simulink model "sldemo_hydrod"  (R2022b)
settings: Solver=ode45  StartTime=0.0  StopTime=0.1  RelTol=1e-3  AbsTol=1e-6
model workspace (MATLAB code in the model file):
  | % Load the initial conditions and initialization data
  | % Using the same MAT file as
  | % sldemo_hydcyl
  | % sldemo_hydcyl4
  | % sldemo_hydrod
  | 
  | load sldemo_hydcyl_data;
undefined symbols (not defined in the file or in its folder): Ac, C2, I, L, M, Qmax
libraries: hydlib x4, simulink x2
(part 1 of 2)
Description:
  | Two Cylinder Model with Load Constraints
  | 
  | In this model, a rigid rod supporting a large mass interconnects two
  | hydraulic actuators. The model eliminates the springs as it applies the
  | piston forces directly to the load. These forces balance the
  | gravitational force and result in both linear and rotational displacement.
  | See two related demos that use the same basic components:
  | 
  | * four cylinder model: sldemo_hydcyl4
  | * single cylinder model: sldemo_hydcyl
settings Model: PacingRate=0.010000  Creator=The MathWorks, Inc.  LastModifiedBy=The MathWorks, Inc.
settings SolverCC: AutoScaleAbsTol=off  AlgebraicLoopSolver=TrustRegion
settings DataIOCC: SaveFormat=Structure  SaveOutput=off  SaveState=on  SaveTime=off  SignalLoggingName=sldemo_hydrod_output
settings OptimizationCC: BlockReduction=off  BooleanDataType=off  ExpressionDepthLimit=2147483647  InitFltsAndDblsToZero=on  LifeSpan=inf  BufferReusableBoundary=off
settings DebuggingCC: AlgebraicLoopMsg=none  SaveWithParameterizedLinksMsg=none  UnderspecifiedInitializationDetection=Classic  MergeDetectMultiDrivingBlocksExec=none  SignalResolutionControl=TryResolveAllWithWarning  MultiTaskDSMMsg=warning  MultiTaskCondExecSysMsg=none  SigSpecEnsureSampleTimeMsg=none  IntegerOverflowMsg=none  FcnCallInpInsideContextMsg=warning  UnconnectedInputMsg=warning  UnconnectedOutputMsg=warning  UnconnectedLineMsg=warning  BusObjectLabelMismatch=none  StateNameClashWarn=warning  SFUnexpectedBacktrackingDiag=warning  SFNoUnconditionalDefaultTransitionDiag=warning  SFExecutionAtInitializationDiag=none  SFMachineParentedDataDiag=warning  IntegerSaturationMsg=none  ArithmeticOperatorsInVariantConditions=warning
settings HardwareCC: ProdBitPerPointer=32  ProdBitPerSizeT=32  ProdBitPerPtrDiffT=32  ProdLargestAtomicFloat=None  ProdIntDivRoundTo=Undefined  ProdEndianess=Unspecified  ProdWordSize=32  ProdHWDeviceType=32-bit Generic  TargetUnknown=on
settings ModelReferenceCC: EnableRefExpFcnMdlSchedulingChecks=on  PropagateSignalLabelsOutOfModel=off
settings SFSimCC: SimUseLocalCustomCode=off  CustomCodeUndefinedFunction=UseInterfaceOnly
settings RTWCC: RTWUseLocalCustomCode=off  DLArmComputeVersion=19.05
settings CodeAppCC: StateflowObjectComments=on
settings GRTTargetCC: TargetFcnLib=ansi_tfl_tmw.mat  TargetLangStandard=C89/C90 (ANSI)  CombineOutputUpdateFcns=off  GRTInterface=on
settings ConfigComp: CovMetricSettings=d  CovSaveCumulativeToWorkspaceVar=on  CovSaveSingleToWorkspaceVar=on  CovExternalEMLEnable=off

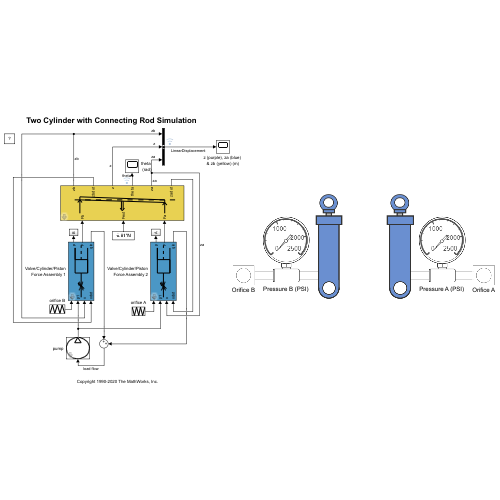
[thumbnail: Simulink's stored preview of the top-level diagram]
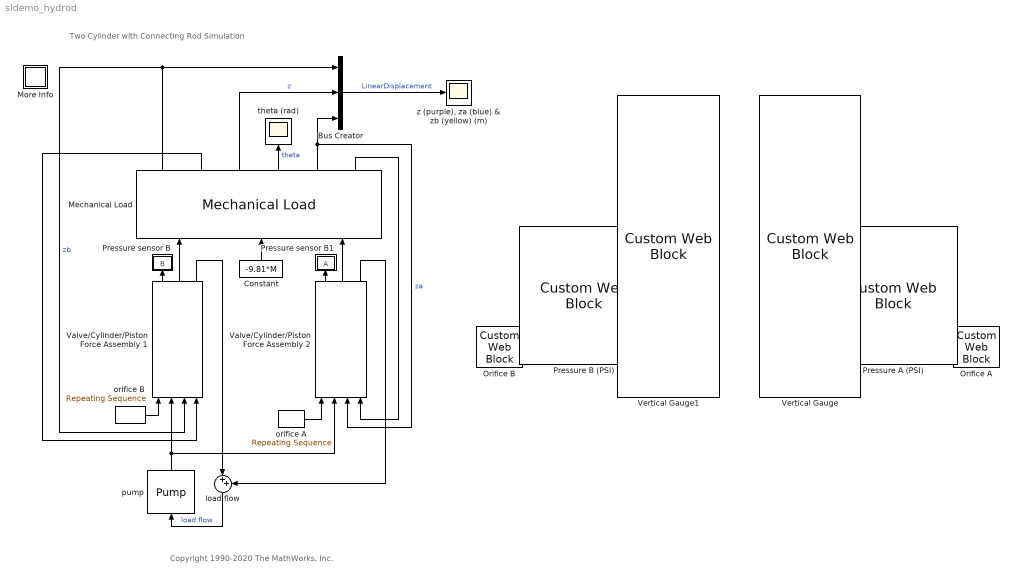
== system sldemo_hydrod ==
  note: Two Cylinder with Connecting Rod Simulation
  note: Copyright 1990-2020 The MathWorks, Inc.
  Bus Creator : BusCreator  Inputs=3
  Constant : Constant  Value=-9.81*M
  Mechanical Load : hydlib/Mechanical Load  L=L  M=M  I=I  zDotName=velocity  zName=displacement  thetaDotName=angular_velocity  thetaName=angular_displacement
  More Info : Subsystem
      settings: OpenFcn=showExample('simulink_general/sldemo_hydrodExample')
      mask Display: disp('?')
  Orifice A : CustomWebBlock  LabelPosition=Hide  ShowInitialText=on  Configuration="{\"type\":\"LinearGauge\",\"settings\":{\"BindingType\":\"signal\",\"aspectRatio\":0.2647058823529412,\"fixedAspectRatio\":\"off\",\"orientation\":\"vertical\",\"value\":0},\"components\":[{\"name\":\"LinearScaleComponent\",\"settings\":{\"bounds\":{\"max\":0.00001,\"min\":0,\"tickInterval\":\"auto\"},\"internalTickHeightScaleFactor\":0.5,\"labelColor\":[250,245,199],\"labelFont\":{\"font\":\"Arial\",\"fontSize\":12},\"labelTransparency\":0,\"needleImage\":{\"size\":[0,0],\"src\":\"\",\"srcOrientation\":\"Right\"},\"needleOffset\":[0,0],\"needleSize\":{\"height\":0,\"width\":0},\"position\":[0.036458333333333336,0.0695754716981132,3.4033018867924527,0.919921875],\"scaleColors\":[],\"scaleColorsSize\":0.2,\"showLabels\":1,\"showMinorTicks\":0,\"showSpanLine\":1,\"showTicks\":1,\"tickColor\":[250,245,200],\"tickTransparency\":0,\"valueBarColor\":[0,0,0],\"valueBarOffset\":0,\"valueBarSize\":0.23,\"valueBarTransparency\":1,\"scaleDirection\":\"BT\",\"referencePoint\":\"auto\",\"labelOffset\":0.05}},{\"name\":\"BackgroundImageComponent\",\"settings\":{\"image\":{\"size\":[0,0],\"src\":\"default\",\"srcOrientation\":null},\"position\":[0,0,1,1],\"scaleMode\":\"0\"}},{\"name\":\"ForegroundImageComponent\",\"settings\":{\"image\":{\"size\":[35,31],\"src\":\"data:image/png;base64,iVBORw0KGgoAAAANSUhEUgAAAp0AAAJbCAYAAACmZC+XAAAACXBIWXMAAA7EAAAOxAGVKw4bAAAAB3RJTUUH5AoDETghXxYhmQAAIABJREFUeJzs3XtwVeW9//HPLqBEKwRNuA3BpAoElJsBArEmgtwsRUkEWqiECug0iMgPM8Fr05wZR0+agwoRLEoqwRJFIKnIMQGEBksgQORmuWMiMFwEJWBruMX1+4OSAzZr7Z2w98rea79fM4xOnmctvtOa/Xz291kXl2EYhgAAAAAf+klDFwAAAADnI3QCAADA5widAAAA8DlCJwAAAHyO0AkAAACfI3QCAADA5widAAAA8DlCJwAAAHyu8fUc7HK5vFUHAAAAAkR93i1EpxMAAAA+R+gEAACAzxE6AQAA ...(+26324 chars)\",\"srcOrientation\":\"vertical\"},\"isForeground\":1,\"position\":[0,0,1,1],\"scaleMode\":\"0\"}}]}"
  Orifice B : CustomWebBlock  LabelPosition=Hide  ShowInitialText=on  Configuration="{\"type\":\"LinearGauge\",\"settings\":{\"BindingType\":\"signal\",\"aspectRatio\":0.2647058823529412,\"fixedAspectRatio\":\"off\",\"orientation\":\"vertical\",\"value\":0},\"components\":[{\"name\":\"LinearScaleComponent\",\"settings\":{\"bounds\":{\"max\":0.00001,\"min\":0,\"tickInterval\":\"auto\"},\"internalTickHeightScaleFactor\":0.5,\"labelColor\":[250,245,199],\"labelFont\":{\"font\":\"Arial\",\"fontSize\":12},\"labelTransparency\":0,\"needleImage\":{\"size\":[0,0],\"src\":\"\",\"srcOrientation\":\"Right\"},\"needleOffset\":[0,0],\"needleSize\":{\"height\":0,\"width\":0},\"position\":[0.036458333333333336,0.0695754716981132,3.4033018867924527,0.919921875],\"scaleColors\":[],\"scaleColorsSize\":0.2,\"showLabels\":1,\"showMinorTicks\":0,\"showSpanLine\":1,\"showTicks\":1,\"tickColor\":[250,245,200],\"tickTransparency\":0,\"valueBarColor\":[0,0,0],\"valueBarOffset\":0,\"valueBarSize\":0.23,\"valueBarTransparency\":1,\"scaleDirection\":\"BT\",\"referencePoint\":\"auto\",\"labelOffset\":0.05}},{\"name\":\"BackgroundImageComponent\",\"settings\":{\"image\":{\"size\":[0,0],\"src\":\"default\",\"srcOrientation\":null},\"position\":[0,0,1,1],\"scaleMode\":\"0\"}},{\"name\":\"ForegroundImageComponent\",\"settings\":{\"image\":{\"size\":[35,31],\"src\":\"data:image/png;base64,iVBORw0KGgoAAAANSUhEUgAAAp0AAAJbCAYAAACmZC+XAAAACXBIWXMAAA7EAAAOxAGVKw4bAAAAB3RJTUUH5AoDETghXxYhmQAAIABJREFUeJzs3XtwVeW9//HPLqBEKwRNuA3BpAoElJsBArEmgtwsRUkEWqiECug0iMgPM8Fr05wZR0+agwoRLEoqwRJFIKnIMQGEBksgQORmuWMiMFwEJWBruMX1+4OSAzZr7Z2w98rea79fM4xOnmctvtOa/Xz291kXl2EYhgAAAAAf+klDFwAAAADnI3QCAADA5widAAAA8DlCJwAAAHyO0AkAAACfI3QCAADA5widAAAA8DlCJwAAAHyu8fUc7HK5vFUHAAAAAkR93i1EpxMAAAA+R+gEAACAzxE6AQAA ...(+26324 chars)\",\"srcOrientation\":\"vertical\"},\"isForeground\":1,\"position\":[0,0,1,1],\"scaleMode\":\"0\"}}]}"
  Pressure A (PSI) : CustomWebBlock  LabelPosition=Hide  ShowInitialText=on  Configuration="{\"type\":\"CircularGauge\",\"settings\":{\"BindingType\":\"signal\",\"aspectRatio\":0.9677819083023544,\"direction\":\"cw\",\"fixedAspectRatio\":\"on\",\"flipLimits\":0,\"orientation\":\"horizontal\",\"value\":0,\"backgroundOffset\":0.14},\"components\":[{\"name\":\"CircularScaleComponent\",\"settings\":{\"bounds\":{\"max\":2500,\"min\":0,\"tickInterval\":\"auto\"},\"direction\":\"cw\",\"flipLimits\":0,\"innerRadius\":0.75,\"internalTickHeightScaleFactor\":1,\"labelColor\":[38,38,38],\"labelFont\":{\"font\":\"Arial\",\"fontSize\":12},\"labelTransparency\":1,\"minorTickHeightScaleFactor\":0.2,\"needleImage\":{\"size\":[79,20],\"src\":\"data:image/svg+xml;base64,PD94bWwgdmVyc2lvbj0iMS4wIiBlbmNvZGluZz0idXRmLTgiPz4KPCEtLSBHZW5lcmF0b3I6IEFkb2JlIElsbHVzdHJhdG9yIDI0LjEuMiwgU1ZHIEV4cG9ydCBQbHVnLUluIC4gU1ZHIFZlcnNpb246IDYuMDAgQnVpbGQgMCkgIC0tPgo8c3ZnIHZlcnNpb249IjEuMSIgaWQ9IkxheWVyXzEiIHhtbG5zPSJodHRwOi8vd3d3LnczLm9yZy8yMDAwL3N2ZyIgeG1sbnM6eGxpbms9Imh0dHA6Ly93d3cudzMub3JnLzE5OTkveGxpbmsiIHg9IjBweCIgeT0iMHB4IgoJIHZpZXdCb3g9IjAgMCA3OC43IDIwIiBzdHlsZT0iZW5hYmxlLWJhY2tncm91bmQ6bmV3IDAgMCA3OC43IDIwOyIgeG1sOnNwYWNlPSJwcmVzZXJ2ZSI+CjxwYXRoIGQ9Ik01My4xLDUuOGwyNS42LTEuNGwtMy41LDVsMy4xLDUuMmwtMjUuNC0xLjNjLTEuNSwyLjMtNC4yLDMuNC02LjksM2MtMi4yLTAuMy00LjItMS43LTUuMi0zLjdMMC45LDEwLjgKCWMtMS4xLDAtMS4yLTEuNi0wLjEtMS43bDM5LjktMi43QzQyLDMuNiw0NSwyLDQ4LDIuNEM1MC4yLDIuOCw1Miw0LDUzLjEsNS44TDUzLjEsNS44eiBNNTMuNywxMS42bDIxLjQsMS4xbC0yLTMuNGwyLjEtMy4xCglMNTMuOCw3LjVDNTMuOSw4LDU0LDguNSw1NCw5LjFDNTQuMSw5LjksNTQsMTAuOCw1My43LDExLjZMNTMuNywxMS42eiBNNDAuMSw4LjJMMTkuMyw5LjVjLTMuOSwwLjMtMy45LDAuMiwwLDAuNGwyMC45LDEKCUM0MCwxMC41LDQwLDEwLDQwLDkuNUM0MCw5LjEsNDAsOC42LDQwLjEsOC4yTDQwLjEsOC4yeiBNNDcuOCw0LjFjLTMuMy0wLjUtNi4yLDIuMS02LjEsNS40YzAsMi42LDEuOSw0LjgsNC41LDUuMQoJYzMuMywwLjUsNi4zLTIuMiw2LjEtNS41QzUyLjIsNi42LDUwLjMsNC41LDQ3LjgsNC4xTDQ3LjgsNC4xeiIvPgo8L3N2Zz4K\"},\"needleOffset\":[0.061149395709068396,0],\"needleOrientation\":-45,\"needleRotation\":180,\"needleSize\":{\"height\":0.1101177838554453,\"width\":0.43719941652583294},\"outerRadius\":0.9,\"position\":[-0.001375,0.1378196848359597,0.7199690002583312,0.75],\"scaleAngle\":270,\"scaleAngleOffset\":135,\"scaleColors\":[],\"scaleColorsSize\":0.2,\"scalePosition\":[0,0,1,1],\"showLabels\":1,\"showMinorTicks\":1,\"showSpanLine\":1,\"showTicks\":1,\"tickColor\":[38,38,38],\"tickTransparency\":1,\"valueBarColor\":[0,114,189],\"valueBarPosition\":[0,0,1,1],\"valueBarSize\":0.2,\"valueBarTransparency\":0,\"scaleDirection\":\"CW\",\"referencePoint\":\"auto\",\"labelRadius\":0.528}},{\"name\":\"BackgroundImageComponent\",\"settings\":{\"image\":{\"size\":[6248,6456],\"src\":\"data:image/svg+xml;base64,PD94bWwgdmVyc2lvbj0iMS4wIiBlbmNvZGluZz0idXRmLTgiPz4KPCEtLSBHZW5lcmF0b3I6IEFkb2JlIElsbHVzdHJhdG9yIDI0LjEuMiwgU1ZHIEV4cG9ydCBQbHVnLUluIC4gU1ZHIFZlcnNpb246IDYuMDAgQnVpbGQgMCkgIC0tPgo8c3ZnIHZlcnNpb249IjEuMSIgaWQ9IkxheWVyXzEiIHhtbG5zOnhvZG09Imh0dHA6Ly93d3cuY29yZWwuY29tL2NvcmVsZHJhdy9vZG0vMjAwMyIKCSB4bWxucz0iaHR0cDovL3d3dy53My5vcmcvMjAwMC9zdmciIHhtbG5zOnhsaW5rPSJodHRwOi8vd3d3LnczLm9yZy8xOTk5L3hsaW5rIiB4 ...(+3504 chars)\",\"srcOrientation\":\"horizontal\"},\"position\":[0,0,1,1],\"scaleMode\":\"0\"}},{\"name\":\"ForegroundImageComponent\",\"settings\":{\"image\":{\"size\":[0,0],\"src\":\"default\",\"srcOrientation\":[]},\"isForeground\":1,\"position\":[0,0,1,1],\"scaleMode\":\"0\"}}]}"
  Pressure B (PSI) : CustomWebBlock  LabelPosition=Hide  ShowInitialText=on  Configuration="{\"type\":\"CircularGauge\",\"settings\":{\"BindingType\":\"signal\",\"aspectRatio\":0.9677819083023544,\"direction\":\"cw\",\"fixedAspectRatio\":\"on\",\"flipLimits\":0,\"orientation\":\"horizontal\",\"value\":0,\"backgroundOffset\":0.14},\"components\":[{\"name\":\"CircularScaleComponent\",\"settings\":{\"bounds\":{\"max\":2500,\"min\":0,\"tickInterval\":\"auto\"},\"direction\":\"cw\",\"flipLimits\":0,\"innerRadius\":0.75,\"internalTickHeightScaleFactor\":1,\"labelColor\":[38,38,38],\"labelFont\":{\"font\":\"Arial\",\"fontSize\":12},\"labelTransparency\":1,\"minorTickHeightScaleFactor\":0.2,\"needleImage\":{\"size\":[79,20],\"src\":\"data:image/svg+xml;base64,PD94bWwgdmVyc2lvbj0iMS4wIiBlbmNvZGluZz0idXRmLTgiPz4KPCEtLSBHZW5lcmF0b3I6IEFkb2JlIElsbHVzdHJhdG9yIDI0LjEuMiwgU1ZHIEV4cG9ydCBQbHVnLUluIC4gU1ZHIFZlcnNpb246IDYuMDAgQnVpbGQgMCkgIC0tPgo8c3ZnIHZlcnNpb249IjEuMSIgaWQ9IkxheWVyXzEiIHhtbG5zPSJodHRwOi8vd3d3LnczLm9yZy8yMDAwL3N2ZyIgeG1sbnM6eGxpbms9Imh0dHA6Ly93d3cudzMub3JnLzE5OTkveGxpbmsiIHg9IjBweCIgeT0iMHB4IgoJIHZpZXdCb3g9IjAgMCA3OC43IDIwIiBzdHlsZT0iZW5hYmxlLWJhY2tncm91bmQ6bmV3IDAgMCA3OC43IDIwOyIgeG1sOnNwYWNlPSJwcmVzZXJ2ZSI+CjxwYXRoIGQ9Ik01My4xLDUuOGwyNS42LTEuNGwtMy41LDVsMy4xLDUuMmwtMjUuNC0xLjNjLTEuNSwyLjMtNC4yLDMuNC02LjksM2MtMi4yLTAuMy00LjItMS43LTUuMi0zLjdMMC45LDEwLjgKCWMtMS4xLDAtMS4yLTEuNi0wLjEtMS43bDM5LjktMi43QzQyLDMuNiw0NSwyLDQ4LDIuNEM1MC4yLDIuOCw1Miw0LDUzLjEsNS44TDUzLjEsNS44eiBNNTMuNywxMS42bDIxLjQsMS4xbC0yLTMuNGwyLjEtMy4xCglMNTMuOCw3LjVDNTMuOSw4LDU0LDguNSw1NCw5LjFDNTQuMSw5LjksNTQsMTAuOCw1My43LDExLjZMNTMuNywxMS42eiBNNDAuMSw4LjJMMTkuMyw5LjVjLTMuOSwwLjMtMy45LDAuMiwwLDAuNGwyMC45LDEKCUM0MCwxMC41LDQwLDEwLDQwLDkuNUM0MCw5LjEsNDAsOC42LDQwLjEsOC4yTDQwLjEsOC4yeiBNNDcuOCw0LjFjLTMuMy0wLjUtNi4yLDIuMS02LjEsNS40YzAsMi42LDEuOSw0LjgsNC41LDUuMQoJYzMuMywwLjUsNi4zLTIuMiw2LjEtNS41QzUyLjIsNi42LDUwLjMsNC41LDQ3LjgsNC4xTDQ3LjgsNC4xeiIvPgo8L3N2Zz4K\"},\"needleOffset\":[0.061149395709068396,0],\"needleOrientation\":-45,\"needleRotation\":180,\"needleSize\":{\"height\":0.1101177838554453,\"width\":0.43719941652583294},\"outerRadius\":0.9,\"position\":[0.0065,0.1379808323486937,0.7195746356833399,0.726],\"scaleAngle\":270,\"scaleAngleOffset\":135,\"scaleColors\":[],\"scaleColorsSize\":0.2,\"scalePosition\":[0,0,1,1],\"showLabels\":1,\"showMinorTicks\":1,\"showSpanLine\":1,\"showTicks\":1,\"tickColor\":[38,38,38],\"tickTransparency\":1,\"valueBarColor\":[0,114,189],\"valueBarPosition\":[0,0,1,1],\"valueBarSize\":0.2,\"valueBarTransparency\":0,\"scaleDirection\":\"CW\",\"referencePoint\":\"auto\",\"labelRadius\":0.528}},{\"name\":\"BackgroundImageComponent\",\"settings\":{\"image\":{\"size\":[6248,6456],\"src\":\"data:image/svg+xml;base64,PD94bWwgdmVyc2lvbj0iMS4wIiBlbmNvZGluZz0idXRmLTgiPz4KPCEtLSBHZW5lcmF0b3I6IEFkb2JlIElsbHVzdHJhdG9yIDI0LjEuMiwgU1ZHIEV4cG9ydCBQbHVnLUluIC4gU1ZHIFZlcnNpb246IDYuMDAgQnVpbGQgMCkgIC0tPgo8c3ZnIHZlcnNpb249IjEuMSIgaWQ9IkxheWVyXzEiIHhtbG5zOnhvZG09Imh0dHA6Ly93d3cuY29yZWwuY29tL2NvcmVsZHJhdy9vZG0vMjAwMyIKCSB4bWxucz0iaHR0cDovL3d3dy53My5vcmcvMjAwMC9zdmciIHhtbG5zOnhsaW5rPSJodHRwOi8vd3d3LnczLm9yZy8xOTk5L3hsaW5rIiB4 ...(+3504 chars)\",\"srcOrientation\":\"horizontal\"},\"position\":[0,0,1,1],\"scaleMode\":\"0\"}},{\"name\":\"ForegroundImageComponent\",\"settings\":{\"image\":{\"size\":[0,0],\"src\":\"default\",\"srcOrientation\":[]},\"isForeground\":1,\"position\":[0,0,1,1],\"scaleMode\":\"0\"}}]}"
  Pressure sensor B : Subsystem
  Pressure sensor B1 : Subsystem
  Valve/Cylinder/Piston Force Assembly 1 : hydlib/Valve//Cylinder//Piston Force Assembly  C1=C1  Ac=Ac  Cd=Cd  rho=rho  V30=V30  beta=Beta  p30=9.81*M/2/Ac  assemblyName=forceLeft
  Valve/Cylinder/Piston Force Assembly 2 : hydlib/Valve//Cylinder//Piston Force Assembly  C1=C1  Ac=Ac  Cd=Cd  rho=rho  V30=V30  beta=Beta  p30=9.81*M/2/Ac  assemblyName=forceRight
  Vertical Gauge : CustomWebBlock  LabelPosition=Hide  ShowInitialText=on  Configuration="{\"type\":\"LinearGauge\",\"settings\":{\"BindingType\":\"signal\",\"aspectRatio\":0.3333333333333333,\"fixedAspectRatio\":\"on\",\"orientation\":\"vertical\",\"value\":0},\"components\":[{\"name\":\"LinearScaleComponent\",\"settings\":{\"bounds\":{\"max\":0.012,\"min\":0,\"tickInterval\":\"auto\"},\"internalTickHeightScaleFactor\":0.5,\"labelColor\":[250,245,199],\"labelFont\":{\"font\":\"Arial\",\"fontSize\":12},\"labelTransparency\":0,\"needleImage\":{\"size\":[192,576],\"src\":\"data:image/svg+xml;base64,PHN2ZyB3aWR0aD0iMTkyIiBoZWlnaHQ9IjU3NiIgeG1sbnM9Imh0dHA6Ly93d3cudzMub3JnLzIwMDAvc3ZnIiB4bWxuczp4bGluaz0iaHR0cDovL3d3dy53My5vcmcvMTk5OS94bGluayIgb3ZlcmZsb3c9ImhpZGRlbiI+PGRlZnM+PGNsaXBQYXRoIGlkPSJjbGlwMCI+PHBhdGggZD0iTTAgMCAxOTIgMCAxOTIgNTc2IDAgNTc2WiIgZmlsbC1ydWxlPSJldmVub2RkIiBjbGlwLXJ1bGU9ImV2ZW5vZGQiLz48L2NsaXBQYXRoPjwvZGVmcz48ZyBjbGlwLXBhdGg9InVybCgjY2xpcDApIj48cmVjdCB4PSIwIiB5PSIwIiB3aWR0aD0iMTkyIiBoZWlnaHQ9IjU3NiIgZmlsbD0iI0ZGRkZGRiIgZmlsbC1vcGFjaXR5PSIwIi8+PHJlY3QgeD0iNzkuNTAwMSIgeT0iMTIxLjUiIHdpZHRoPSIzMiIgaGVpZ2h0PSI0NTIiIHN0cm9rZT0iIzAwMDAwMCIgc3Ryb2tlLXdpZHRoPSI3IiBzdHJva2UtbWl0ZXJsaW1pdD0iOCIgZmlsbD0iI0E2QTZBNiIvPjxwYXRoIGQ9Ik00MC41MDAxIDU4QzQwLjUwMDEgMjcuOTAwNSA2NC45MDA1IDMuNTAwMDUgOTUgMy41MDAwNSAxMjUuMSAzLjUwMDA1IDE0OS41IDI3LjkwMDUgMTQ5LjUgNTggMTQ5LjUgODguMDk5NiAxMjUuMSAxMTIuNSA5NSAxMTIuNSA2NC45MDA1IDExMi41IDQwLjUwMDEgODguMDk5NiA0MC41MDAxIDU4WiIgc3Ryb2tlPSIjMDAwMDAwIiBzdHJva2Utd2lkdGg9IjUiIHN0cm9rZS1taXRlcmxpbWl0PSI4IiBmaWxsPSIjNDQ3MkM0IiBmaWxsLXJ1bGU9ImV2ZW5vZGQiLz48cmVjdCB4PSI2MS41MDAxIiB5PSIxMDEuNSIgd2lkdGg9IjY5IiBoZWlnaHQ9IjIwIiBzdHJva2U9IiMwMDAwMDAiIHN0cm9rZS13aWR0aD0iNyIgc3Ryb2tlLW1pdGVybGltaXQ9IjgiIGZpbGw9IiM0NDcyQzQiLz48cGF0aCBkPSJNNjQuNTAwMSA1NS4wMDAxQzY0LjUwMDEgMzguMTU1NCA3OC4xNTU0IDI0LjUwMDEgOTUuMDAwMSAyNC41MDAxIDExMS44NDUgMjQuNTAwMSAxMjUuNSAzOC4xNTU0IDEyNS41IDU1LjAwMDEgMTI1LjUgNzEuODQ0NyAxMTEuODQ1IDg1LjUwMDEgOTUuMDAwMSA4NS41MDAxIDc4LjE1NTQgODUuNTAwMSA2NC41MDAxIDcxLjg0NDcgNjQuNTAwMSA1NS4wMDAxWiIgc3Ryb2tlPSIjMDAwMDAwIiBzdHJva2Utd2lkdGg9IjUiIHN0cm9rZS1taXRlcmxpbWl0PSI4IiBmaWxsPSIjRkZGRkZGIiBmaWxsLXJ1bGU9ImV2ZW5vZGQiLz48L2c+PC9zdmc+\",\"srcOrientation\":\"Right\"},\"needleOffset\":[-0.0371900826446281,-0.19204801200300076],\"needleSize\":{\"height\":0.587378640776699,\"width\":0.6125919117647058},\"position\":[0.2412014563106796,0.2516084558823529,0.5994944852941176,0.39638956310679613],\"scaleColors\":[],\"scaleColorsSize\":0.2,\"showLabels\":1,\"showMinorTicks\":0,\"showSpanLine\":1,\"showTicks\":1,\"tickColor\":[250,245,200],\"tickTransparency\":0,\"valueBarColor\":[23,89,176],\"valueBarOffset\":0,\"valueBarSize\":0.23,\"valueBarTransparency\":0,\"scaleDirection\":\"BT\",\"referencePoint\":\"auto\",\"labelOffset\":0.05}},{\"name\":\"BackgroundImageComponent\",\"settings\":{\"image\":{\"size\":[0,0],\"src\":\"default\",\"srcOrientation\":null},\"position\":[0,0,1,1],\"scaleMode\":\"0\"}},{\"name\":\"ForegroundImageComponent\",\"settings\":{\"image\":{\"size\":[288,864],\"src\":\"data:image/svg+xml;base64,PHN2ZyB3aWR0aD0iMjg4IiBoZWlnaHQ9Ijg2NCIgeG1sbnM9Imh0dHA6Ly93d3cudzMub3JnLzIwMDAvc3ZnIiB4bWxuczp4bGluaz0iaHR0cDovL3d3dy53My5vcmcvMTk5OS94bGluayIgb3ZlcmZsb3c9ImhpZGRlbiI+PGRlZnM+PGNsaXBQYXRoIGlkPSJjbGlwMCI+PHBhdGggZD0iTTAgMCAyODggMCAyODggODY0IDAgODY0WiIgZmlsbC1ydWxlPSJldmVub2RkIiBjbGlwLXJ1bGU9ImV2ZW5vZGQiLz48L2NsaXBQYXRoPjwvZGVmcz48ZyBjbGlwLXBhdGg9InVybCgjY2xpcDApIj48cmVjdCB4PSIwIiB5PSIwIiB3aWR0aD0iMjg4IiBoZWlnaHQ9Ijg2NCIgZmlsbD0iI0ZGRkZGRiIgZmlsbC1vcGFjaXR5PSIwIi8+PHJlY3QgeD0iODYuNTAwMSIgeT0iNDMyLjUiIHdpZHRoPSIxMTYiIGhlaWdodD0iMzY3IiBzdHJva2U9IiMwMDAwMDAiIHN0cm9rZS13aWR0aD0iNyIgc3Ryb2tlLW1pdGVybGltaXQ9IjgiIGZpbGw9IiM0NDcyQzQiLz48cmVjdCB4PSI3Mi41MDAxIiB5PSIzODMuNSIgd2lkdGg9IjE0NiIgaGVpZ2h0PSI0OSIgc3Ryb2tlPSIjMDAwMDAwIiBzdHJva2Utd2lkdGg9IjciIHN0cm9rZS1taXRlcmxpbWl0PSI4IiBmaWxsPSIjNDQ3MkM0Ii8+PHBhdGggZD0iTTIwMi41IDc5MkMyMDIuNSA4MjMuNzU3IDE3Ni41MzMgODQ5LjUgMTQ0LjUgODQ5LjUgMTEyLjcyMSA4NDkuNSA4Ni44NTk1IDgyNC4xNDcgODYuNTAzNyA3OTIuNjQ0TDE0NC41IDc5MloiIHN0cm9rZT0iIzAwMDAwMCIgc3Ryb2tlLXdpZHRoPSI3IiBzdHJva2UtbWl0ZXJsaW1pdD0iOCIgZmlsbD0iIzQ0NzJDNCIgZmlsbC1ydWxlPSJldmVub2RkIi8+PHJlY3QgeD0iOTEiIHk9Ijc0NyIgd2lkdGg9IjEwOCIgaGVpZ2h0PSI0OSIgZmlsbD0iIzQ0NzJDNCIvPjxwYXRoIGQ9Ik0xMDkuNSA3OTEuNUMxMDkuNSA3NzEuNjE4IDEyNS42MTggNzU1LjUgMTQ1LjUgNzU1LjUgMTY1LjM4MiA3NTUuNSAxODEuNSA3NzEuNjE4IDE4MS41IDc5MS41IDE4MS41IDgxMS4zODIgMTY1LjM4MiA4MjcuNSAxNDUuNSA4MjcuNSAxMjUuNjE4IDgyNy41IDEwOS41IDgxMS4zODIgMTA5LjUgNzkxLjVaIiBzdHJva2U9IiMwMDAwMDAiIHN0cm9rZS13aWR0aD0iNSIgc3Ryb2tlLW1pdGVybGltaXQ9IjgiIGZpbGw9IiNGRkZGRkYiIGZpbGwtcnVsZT0iZXZlbm9kZCIvPjwvZz48L3N2Zz4=\",\"srcOrientation\":\"vertical\"},\"isForeground\":1,\"position\":[0,0,1,1],\"scaleMode\":\"0\"}}]}"
  Vertical Gauge1 : CustomWebBlock  LabelPosition=Hide  ShowInitialText=on  Configuration="{\"type\":\"LinearGauge\",\"settings\":{\"BindingType\":\"signal\",\"aspectRatio\":0.3333333333333333,\"fixedAspectRatio\":\"on\",\"orientation\":\"vertical\",\"value\":0},\"components\":[{\"name\":\"LinearScaleComponent\",\"settings\":{\"bounds\":{\"max\":0.012,\"min\":0,\"tickInterval\":\"auto\"},\"internalTickHeightScaleFactor\":0.5,\"labelColor\":[250,245,199],\"labelFont\":{\"font\":\"Arial\",\"fontSize\":12},\"labelTransparency\":0,\"needleImage\":{\"size\":[192,576],\"src\":\"data:image/svg+xml;base64,PHN2ZyB3aWR0aD0iMTkyIiBoZWlnaHQ9IjU3NiIgeG1sbnM9Imh0dHA6Ly93d3cudzMub3JnLzIwMDAvc3ZnIiB4bWxuczp4bGluaz0iaHR0cDovL3d3dy53My5vcmcvMTk5OS94bGluayIgb3ZlcmZsb3c9ImhpZGRlbiI+PGRlZnM+PGNsaXBQYXRoIGlkPSJjbGlwMCI+PHBhdGggZD0iTTAgMCAxOTIgMCAxOTIgNTc2IDAgNTc2WiIgZmlsbC1ydWxlPSJldmVub2RkIiBjbGlwLXJ1bGU9ImV2ZW5vZGQiLz48L2NsaXBQYXRoPjwvZGVmcz48ZyBjbGlwLXBhdGg9InVybCgjY2xpcDApIj48cmVjdCB4PSIwIiB5PSIwIiB3aWR0aD0iMTkyIiBoZWlnaHQ9IjU3NiIgZmlsbD0iI0ZGRkZGRiIgZmlsbC1vcGFjaXR5PSIwIi8+PHJlY3QgeD0iNzkuNTAwMSIgeT0iMTIxLjUiIHdpZHRoPSIzMiIgaGVpZ2h0PSI0NTIiIHN0cm9rZT0iIzAwMDAwMCIgc3Ryb2tlLXdpZHRoPSI3IiBzdHJva2UtbWl0ZXJsaW1pdD0iOCIgZmlsbD0iI0E2QTZBNiIvPjxwYXRoIGQ9Ik00MC41MDAxIDU4QzQwLjUwMDEgMjcuOTAwNSA2NC45MDA1IDMuNTAwMDUgOTUgMy41MDAwNSAxMjUuMSAzLjUwMDA1IDE0OS41IDI3LjkwMDUgMTQ5LjUgNTggMTQ5LjUgODguMDk5NiAxMjUuMSAxMTIuNSA5NSAxMTIuNSA2NC45MDA1IDExMi41IDQwLjUwMDEgODguMDk5NiA0MC41MDAxIDU4WiIgc3Ryb2tlPSIjMDAwMDAwIiBzdHJva2Utd2lkdGg9IjUiIHN0cm9rZS1taXRlcmxpbWl0PSI4IiBmaWxsPSIjNDQ3MkM0IiBmaWxsLXJ1bGU9ImV2ZW5vZGQiLz48cmVjdCB4PSI2MS41MDAxIiB5PSIxMDEuNSIgd2lkdGg9IjY5IiBoZWlnaHQ9IjIwIiBzdHJva2U9IiMwMDAwMDAiIHN0cm9rZS13aWR0aD0iNyIgc3Ryb2tlLW1pdGVybGltaXQ9IjgiIGZpbGw9IiM0NDcyQzQiLz48cGF0aCBkPSJNNjQuNTAwMSA1NS4wMDAxQzY0LjUwMDEgMzguMTU1NCA3OC4xNTU0IDI0LjUwMDEgOTUuMDAwMSAyNC41MDAxIDExMS44NDUgMjQuNTAwMSAxMjUuNSAzOC4xNTU0IDEyNS41IDU1LjAwMDEgMTI1LjUgNzEuODQ0NyAxMTEuODQ1IDg1LjUwMDEgOTUuMDAwMSA4NS41MDAxIDc4LjE1NTQgODUuNTAwMSA2NC41MDAxIDcxLjg0NDcgNjQuNTAwMSA1NS4wMDAxWiIgc3Ryb2tlPSIjMDAwMDAwIiBzdHJva2Utd2lkdGg9IjUiIHN0cm9rZS1taXRlcmxpbWl0PSI4IiBmaWxsPSIjRkZGRkZGIiBmaWxsLXJ1bGU9ImV2ZW5vZGQiLz48L2c+PC9zdmc+\",\"srcOrientation\":\"Right\"},\"needleOffset\":[-0.0371900826446281,-0.19204801200300076],\"needleSize\":{\"height\":0.587378640776699,\"width\":0.6125919117647058},\"position\":[0.2412014563106796,0.2516084558823529,0.5994944852941176,0.39638956310679613],\"scaleColors\":[],\"scaleColorsSize\":0.2,\"showLabels\":1,\"showMinorTicks\":0,\"showSpanLine\":1,\"showTicks\":1,\"tickColor\":[250,245,200],\"tickTransparency\":0,\"valueBarColor\":[23,89,176],\"valueBarOffset\":0,\"valueBarSize\":0.23,\"valueBarTransparency\":0,\"scaleDirection\":\"BT\",\"referencePoint\":\"auto\",\"labelOffset\":0.05}},{\"name\":\"BackgroundImageComponent\",\"settings\":{\"image\":{\"size\":[0,0],\"src\":\"default\",\"srcOrientation\":null},\"position\":[0,0,1,1],\"scaleMode\":\"0\"}},{\"name\":\"ForegroundImageComponent\",\"settings\":{\"image\":{\"size\":[288,864],\"src\":\"data:image/svg+xml;base64,PHN2ZyB3aWR0aD0iMjg4IiBoZWlnaHQ9Ijg2NCIgeG1sbnM9Imh0dHA6Ly93d3cudzMub3JnLzIwMDAvc3ZnIiB4bWxuczp4bGluaz0iaHR0cDovL3d3dy53My5vcmcvMTk5OS94bGluayIgb3ZlcmZsb3c9ImhpZGRlbiI+PGRlZnM+PGNsaXBQYXRoIGlkPSJjbGlwMCI+PHBhdGggZD0iTTAgMCAyODggMCAyODggODY0IDAgODY0WiIgZmlsbC1ydWxlPSJldmVub2RkIiBjbGlwLXJ1bGU9ImV2ZW5vZGQiLz48L2NsaXBQYXRoPjwvZGVmcz48ZyBjbGlwLXBhdGg9InVybCgjY2xpcDApIj48cmVjdCB4PSIwIiB5PSIwIiB3aWR0aD0iMjg4IiBoZWlnaHQ9Ijg2NCIgZmlsbD0iI0ZGRkZGRiIgZmlsbC1vcGFjaXR5PSIwIi8+PHJlY3QgeD0iODYuNTAwMSIgeT0iNDMyLjUiIHdpZHRoPSIxMTYiIGhlaWdodD0iMzY3IiBzdHJva2U9IiMwMDAwMDAiIHN0cm9rZS13aWR0aD0iNyIgc3Ryb2tlLW1pdGVybGltaXQ9IjgiIGZpbGw9IiM0NDcyQzQiLz48cmVjdCB4PSI3Mi41MDAxIiB5PSIzODMuNSIgd2lkdGg9IjE0NiIgaGVpZ2h0PSI0OSIgc3Ryb2tlPSIjMDAwMDAwIiBzdHJva2Utd2lkdGg9IjciIHN0cm9rZS1taXRlcmxpbWl0PSI4IiBmaWxsPSIjNDQ3MkM0Ii8+PHBhdGggZD0iTTIwMi41IDc5MkMyMDIuNSA4MjMuNzU3IDE3Ni41MzMgODQ5LjUgMTQ0LjUgODQ5LjUgMTEyLjcyMSA4NDkuNSA4Ni44NTk1IDgyNC4xNDcgODYuNTAzNyA3OTIuNjQ0TDE0NC41IDc5MloiIHN0cm9rZT0iIzAwMDAwMCIgc3Ryb2tlLXdpZHRoPSI3IiBzdHJva2UtbWl0ZXJsaW1pdD0iOCIgZmlsbD0iIzQ0NzJDNCIgZmlsbC1ydWxlPSJldmVub2RkIi8+PHJlY3QgeD0iOTEiIHk9Ijc0NyIgd2lkdGg9IjEwOCIgaGVpZ2h0PSI0OSIgZmlsbD0iIzQ0NzJDNCIvPjxwYXRoIGQ9Ik0xMDkuNSA3OTEuNUMxMDkuNSA3NzEuNjE4IDEyNS42MTggNzU1LjUgMTQ1LjUgNzU1LjUgMTY1LjM4MiA3NTUuNSAxODEuNSA3NzEuNjE4IDE4MS41IDc5MS41IDE4MS41IDgxMS4zODIgMTY1LjM4MiA4MjcuNSAxNDUuNSA4MjcuNSAxMjUuNjE4IDgyNy41IDEwOS41IDgxMS4zODIgMTA5LjUgNzkxLjVaIiBzdHJva2U9IiMwMDAwMDAiIHN0cm9rZS13aWR0aD0iNSIgc3Ryb2tlLW1pdGVybGltaXQ9IjgiIGZpbGw9IiNGRkZGRkYiIGZpbGwtcnVsZT0iZXZlbm9kZCIvPjwvZz48L3N2Zz4=\",\"srcOrientation\":\"vertical\"},\"isForeground\":1,\"position\":[0,0,1,1],\"scaleMode\":\"0\"}}]}"
  load flow : Sum  Inputs=|++  InputSameDT=on  SaturateOnIntegerOverflow=on  OutDataTypeStr=Inherit: Same as first input
  orifice A : simulink/Sources/Repeating Sequence  rep_seq_t="[0  0.1  0.2]/10"  rep_seq_y=[1 0 1]*1e-5
  orifice B : simulink/Sources/Repeating Sequence  rep_seq_t=[0 0.1 0.2]/10  rep_seq_y=[0 1 0]*1e-5
  pump : hydlib/Pump  t="[0        .04]"  Qpump=Qmax*[1 1]  p10=9.81*M/2/Ac  C2=C2/10
  theta (rad) : Scope
  "z (purple), za (blue) & zb (yellow) (m)" : Scope
  wires:
  Mechanical Load/1 -> Valve/Cylinder/Piston Force Assembly 1/3, Bus Creator/1  "zb"
  Mechanical Load/5 -> Valve/Cylinder/Piston Force Assembly 2/3, Bus Creator/3  "za"
  Mechanical Load/3 -> Bus Creator/2  "z"
  Mechanical Load/4 -> theta (rad)/1  "theta"
  Constant/1 -> Mechanical Load/2
  Bus Creator/1 -> "z (purple), za (blue) & zb (yellow) (m)"/1  "LinearDisplacement"
  Valve/Cylinder/Piston Force Assembly 2/2 -> Mechanical Load/3
  Mechanical Load/6 -> Valve/Cylinder/Piston Force Assembly 2/4
  orifice A/1 -> Valve/Cylinder/Piston Force Assembly 2/1
  Valve/Cylinder/Piston Force Assembly 2/1 -> Pressure sensor B1/1(A)
  Valve/Cylinder/Piston Force Assembly 1/2 -> Mechanical Load/1
  Mechanical Load/2 -> Valve/Cylinder/Piston Force Assembly 1/4
  orifice B/1 -> Valve/Cylinder/Piston Force Assembly 1/1
  Valve/Cylinder/Piston Force Assembly 1/1 -> Pressure sensor B/1(B)
  pump/1 -> Valve/Cylinder/Piston Force Assembly 1/2, Valve/Cylinder/Piston Force Assembly 2/2
  load flow/1 -> pump/1  "load flow"
  Valve/Cylinder/Piston Force Assembly 2/3 -> load flow/2
  Valve/Cylinder/Piston Force Assembly 1/3 -> load flow/1
